simulink model "fine_delay_core"  (R2012b)
settings: Solver=ode45  StartTime=0.0  StopTime=10.0  RelTol=1e-3
libraries: xbsIndex_r4 x410, casper_library_misc x16, casper_library_multipliers x8
(part 1 of 4)
settings Model: Creator=jack  LastModifiedBy=jack

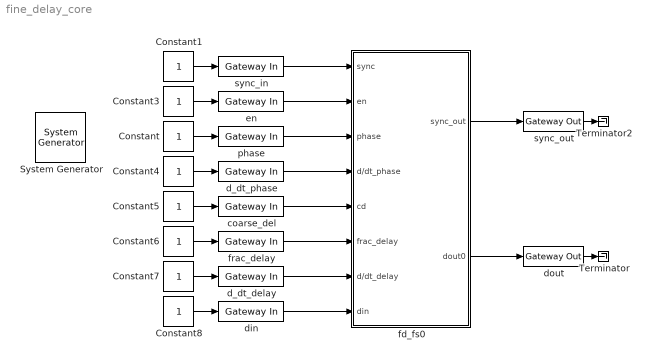
== system fine_delay_core ==
  " System Generator" : xbsIndex_r4/ System Generator  Tag=genX  xilinxfamily=virtex6  part=xc6vsx475t  speed=-1  package=ff1759  synthesis_tool=XST  clock_wrapper=Clock Enables  directory=./fine_delay_core  proj_type=Project Navigator  Synth_file=XST Defaults  Impl_file=ISE Defaults  testbench=off  simulink_period=1  sysclk_period=10  dcm_input_clock_period=10  incr_netlist=off  trim_vbits=Everywhere in SubSystem  dbl_ovrd=According to Block Masks  core_generation=According to Block Masks  run_coregen=off  deprecated_control=off  eval_field=0  block_type=sysgen
  Constant{,1,3..8} (8 alike) : Constant
  Terminator : Terminator
  Terminator2 : Terminator
  coarse_del : xbsIndex_r4/Gateway In  gui_display_data_type=Fixed-point  arith_type=Unsigned  n_bits=15  bin_pt=0  preci_type=Single  exp_width=8  frac_width=24  quantization="Round  (unbiased: +/- Inf)"  overflow=Saturate  period=1  dbl_ovrd=off  timing_constraint=None  locs_specified=off  LOCs={}  UseAsADC=off  ADCChannel='1'  inherit_from_input=off  hdl_port=on  block_type=gatewayin
  d_dt_delay : xbsIndex_r4/Gateway In  gui_display_data_type=Fixed-point  arith_type=Unsigned  n_bits=16  bin_pt=0  preci_type=Single  exp_width=8  frac_width=24  quantization="Round  (unbiased: +/- Inf)"  overflow=Saturate  period=1  dbl_ovrd=off  timing_constraint=None  locs_specified=off  LOCs={}  UseAsADC=off  ADCChannel='1'  inherit_from_input=off  hdl_port=on  block_type=gatewayin
  d_dt_phase : xbsIndex_r4/Gateway In  gui_display_data_type=Fixed-point  arith_type=Unsigned  n_bits=16  bin_pt=0  preci_type=Single  exp_width=8  frac_width=24  quantization="Round  (unbiased: +/- Inf)"  overflow=Saturate  period=1  dbl_ovrd=off  timing_constraint=None  locs_specified=off  LOCs={}  UseAsADC=off  ADCChannel='1'  inherit_from_input=off  hdl_port=on  block_type=gatewayin
  din : xbsIndex_r4/Gateway In  gui_display_data_type=Fixed-point  arith_type=Unsigned  n_bits=8*36  bin_pt=0  preci_type=Single  exp_width=8  frac_width=24  quantization="Round  (unbiased: +/- Inf)"  overflow=Saturate  period=1  dbl_ovrd=off  timing_constraint=None  locs_specified=off  LOCs={}  UseAsADC=off  ADCChannel='1'  inherit_from_input=off  hdl_port=on  block_type=gatewayin
  dout : xbsIndex_r4/Gateway Out  inherit_from_input=off  hdl_port=on  timing_constraint=None  locs_specified=off  LOCs={}  UseAsDAC=off  DACChannel='1'  block_type=gatewayout
  en : xbsIndex_r4/Gateway In  gui_display_data_type=Boolean  arith_type=Boolean  n_bits=16  bin_pt=14  preci_type=Single  exp_width=8  frac_width=24  quantization="Round  (unbiased: +/- Inf)"  overflow=Saturate  period=1  dbl_ovrd=off  timing_constraint=None  locs_specified=off  LOCs={}  UseAsADC=off  ADCChannel='1'  inherit_from_input=off  hdl_port=on  block_type=gatewayin
  fd_fs0 : Subsystem
  frac_delay : xbsIndex_r4/Gateway In  gui_display_data_type=Fixed-point  arith_type=Unsigned  n_bits=16  bin_pt=0  preci_type=Single  exp_width=8  frac_width=24  quantization="Round  (unbiased: +/- Inf)"  overflow=Saturate  period=1  dbl_ovrd=off  timing_constraint=None  locs_specified=off  LOCs={}  UseAsADC=off  ADCChannel='1'  inherit_from_input=off  hdl_port=on  block_type=gatewayin
  phase : xbsIndex_r4/Gateway In  gui_display_data_type=Fixed-point  arith_type=Unsigned  n_bits=16  bin_pt=0  preci_type=Single  exp_width=8  frac_width=24  quantization="Round  (unbiased: +/- Inf)"  overflow=Saturate  period=1  dbl_ovrd=off  timing_constraint=None  locs_specified=off  LOCs={}  UseAsADC=off  ADCChannel='1'  inherit_from_input=off  hdl_port=on  block_type=gatewayin
  sync_in : xbsIndex_r4/Gateway In  gui_display_data_type=Boolean  arith_type=Boolean  n_bits=16  bin_pt=14  preci_type=Single  exp_width=8  frac_width=24  quantization="Round  (unbiased: +/- Inf)"  overflow=Saturate  period=1  dbl_ovrd=off  timing_constraint=None  locs_specified=off  LOCs={}  UseAsADC=off  ADCChannel='1'  inherit_from_input=off  hdl_port=on  block_type=gatewayin
  sync_out : xbsIndex_r4/Gateway Out  inherit_from_input=off  hdl_port=on  timing_constraint=None  locs_specified=off  LOCs={}  UseAsDAC=off  DACChannel='1'  block_type=gatewayout
  wires:
  fd_fs0/1(sync_out) -> sync_out/1
  fd_fs0/2(dout0) -> dout/1
  sync_in/1 -> fd_fs0/1(sync)
  Constant/1 -> phase/1
  Constant1/1 -> sync_in/1
  dout/1 -> Terminator/1
  sync_out/1 -> Terminator2/1
  Constant3/1 -> en/1
  en/1 -> fd_fs0/2(en)
  phase/1 -> fd_fs0/3(phase)
  Constant4/1 -> d_dt_phase/1
  d_dt_phase/1 -> fd_fs0/4(d/dt_phase)
  Constant6/1 -> frac_delay/1
  Constant8/1 -> din/1
  Constant7/1 -> d_dt_delay/1
  Constant5/1 -> coarse_del/1
  din/1 -> fd_fs0/8(din)
  d_dt_delay/1 -> fd_fs0/7(d/dt_delay)
  coarse_del/1 -> fd_fs0/5(cd)
  frac_delay/1 -> fd_fs0/6(frac_delay)

== system fine_delay_core/fd_fs0 ==
  sync : Inport
  en : Inport  Port=2
  phase : Inport  Port=3
  d/dt_phase : Inport  Port=4
  cd : Inport  Port=5
  frac_delay : Inport  Port=6
  d/dt_delay : Inport  Port=7
  din : Inport  Port=8
  Concat : xbsIndex_r4/Concat  num_inputs=2  dbl_ovrd=off  block_type=concat
  Constant53 : xbsIndex_r4/Constant  const=0  gui_display_data_type=Fixed-point  arith_type=Boolean  n_bits=1  bin_pt=0  preci_type=Single  exp_width=8  frac_width=24  explicit_period=off  period=1  equ=P=C  opselect=C  inp2=PCIN>>17  opr=+  inp1=P  carry=CIN  dbl_ovrd=off  block_type=constant
      settings: block_version=11.4
  Terminator59 : Terminator
  Terminator60 : Terminator
  delay_gen0 : Subsystem  mask{fft_len=12, phase_bits=16, max_fringe_rate=23, min_fringe_rate=38, delay_bits=16+15, delay_bin_pt=16, max_delay_rate=23, min_delay_rate=38, add_latency=1, lookup_bits=11, cd_bits=15}
      mask prompts: fft_len "FFT size (2^?)"; phase_bits "Input phase resolution (2*pi/2^? radians)"; max_fringe_rate "Max fringe update rate (1/2^? radians/sample)"; min_fringe_rate "Min (non-zero) fringe rate (1/2^? radians/sample)"; delay_bits "Input delay resolution (bits)"; delay_bin_pt "Input delay binary point"; max_delay_rate "Max delay update rate (1/2^? samples/sample)"; min_delay_rate "Min (non-zero) delay update rate (1/2^? samples/sample)"; add_latency "Add latency"; lookup_bits "DDS lookup table resolution (2*pi/2^?)"; cd_bits "Coarse delay range (2^? bits)"
  fd_fs0 : Subsystem  mask{lookup_bit_width=11, data_bit_width=18, fft_len=10, mix_bits=18, bram_latency=3, mult_latency=2, add_latency=1, conv_latency=3}
      mask prompts: lookup_bit_width "Phase resolution (2pi/2^?)"; data_bit_width "Data bit width"; fft_len "FFT length 2^?"; mix_bits "Mixing product bit width"; bram_latency "BRAM latency"; mult_latency "Mult latency"; add_latency "Adder latency"; conv_latency "Convert latency"
      mask init:
      | for i=[0:7]
      |     set_param([gcb,'/rotate',num2str(i),'/sincos0'], ...
      |         'bit_width', 'mix_bits', ...
      |         'bram_latency', 'bram_latency', ...
      |         'depth_bits', 'lookup_bit_width');
      | end
  sync_out : Outport
  dout0 : Outport  Port=2
  wires:
  fd_fs0/1(sync_out) -> sync_out/1
  delay_gen0/3(cd_o) -> Terminator60/1
  delay_gen0/2(en_out) -> Terminator59/1
  delay_gen0/5(slope_out) -> fd_fs0/3(a1)
  delay_gen0/4(phase_out) -> fd_fs0/2(a0)
  delay_gen0/1(sync_out) -> fd_fs0/1(sync_in)
  sync/1 -> delay_gen0/1(sync_in)
  en/1 -> delay_gen0/2(en)
  phase/1 -> delay_gen0/3(phase)
  d/dt_phase/1 -> delay_gen0/4(d/dt_phase)
  din/1 -> delay_gen0/7(din)
  d/dt_delay/1 -> delay_gen0/6(d/dt_delay)
  cd/1 -> Concat/1
  frac_delay/1 -> Concat/2
  Concat/1 -> delay_gen0/5(delay)
  Constant53/1 -> delay_gen0/8(invert_slope)
  delay_gen0/6(dout) -> fd_fs0/4(din)
  delay_gen0/7(idx_d0) -> fd_fs0/5(idx_din0)
  delay_gen0/8(idx_d1) -> fd_fs0/6(idx_din1)
  delay_gen0/9(idx_d2) -> fd_fs0/7(idx_din2)
  delay_gen0/10(idx_d3) -> fd_fs0/8(idx_din3)
  delay_gen0/11(idx_d4) -> fd_fs0/9(idx_din4)
  delay_gen0/12(idx_d5) -> fd_fs0/10(idx_din5)
  delay_gen0/13(idx_d6) -> fd_fs0/11(idx_din6)
  delay_gen0/14(idx_d7) -> fd_fs0/12(idx_din7)
  fd_fs0/2(dout) -> dout0/1

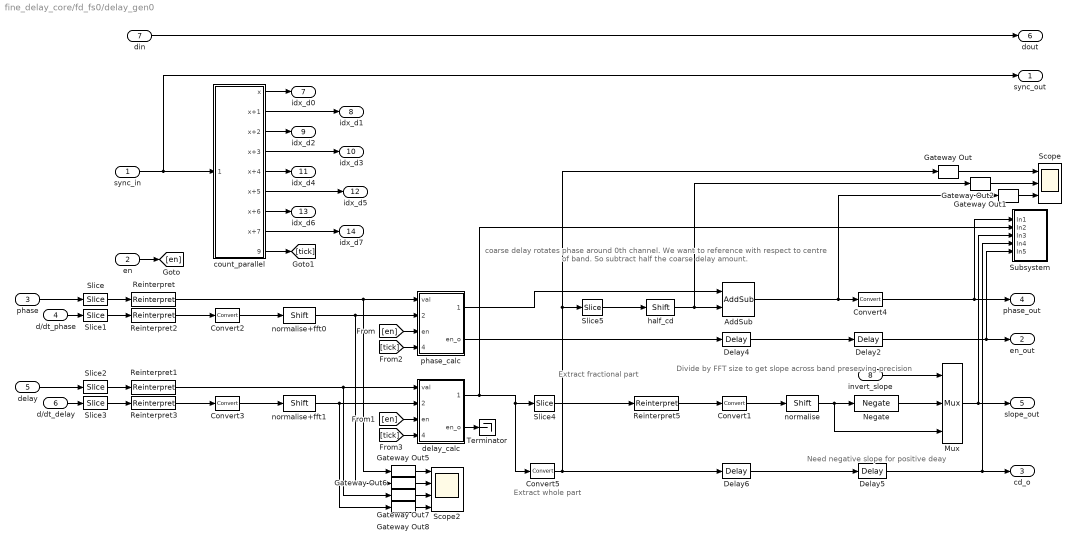
== system fine_delay_core/fd_fs0/delay_gen0 ==
  note: Need negative slope
      | for positive deay
  note: Divide by FFT size
      | to get slope
      | across band
      | preserving precision
  note: Extract whole part
  note: Extract fractional part
  note: coarse delay rotates phase around 0th
      | channel. We want to reference with respect to
      | centre of band. So subtract half the coarse
      | delay amount.
  sync_in : Inport
  en : Inport  Port=2
  phase : Inport  Port=3
  d/dt_phase : Inport  Port=4
  delay : Inport  Port=5
  d/dt_delay : Inport  Port=6
  din : Inport  Port=7
  invert_slope : Inport  Port=8
  AddSub : xbsIndex_r4/AddSub  mode=Addition  use_carryin=off  use_carryout=off  en=off  latency=0  precision=Full  arith_type=Unsigned  n_bits=16  bin_pt=14  quantization=Truncate  overflow=Wrap  dbl_ovrd=off  use_behavioral_HDL=off  hw_selection=Fabric  pipelined=off  block_type=addsub
  Convert1 : xbsIndex_r4/Convert  gui_display_data_type=Fixed-point  arith_type="Signed  (2's comp)"  n_bits=lookup_bits + fft_len  bin_pt=lookup_bits + fft_len -1  float_type=Single  exp_bits=8  fraction_bits=24  quantization="Round  (unbiased: +/- Inf)"  overflow=Wrap  en=off  latency=1  dbl_ovrd=off  pipeline=on  block_type=convert
      settings: block_version=10.1.3
  Convert2 : xbsIndex_r4/Convert  gui_display_data_type=Fixed-point  arith_type="Signed  (2's comp)"  n_bits=min_fringe_rate-fft_len+1  bin_pt=min_fringe_rate-fft_len  float_type=Single  exp_bits=8  fraction_bits=24  quantization=Truncate  overflow=Wrap  en=off  latency=0  dbl_ovrd=off  pipeline=on  block_type=convert
      settings: block_version=10.1.3
  Convert3 : xbsIndex_r4/Convert  gui_display_data_type=Fixed-point  arith_type="Signed  (2's comp)"  n_bits=min_delay_rate-fft_len+1  bin_pt=min_delay_rate-fft_len  float_type=Single  exp_bits=8  fraction_bits=24  quantization=Truncate  overflow=Wrap  en=off  latency=0  dbl_ovrd=off  pipeline=on  block_type=convert
      settings: block_version=10.1.3
  Convert4 : xbsIndex_r4/Convert  gui_display_data_type=Fixed-point  arith_type="Signed  (2's comp)"  n_bits=max(phase_bits, min_fringe_rate-fft_len+1)  bin_pt=max(phase_bits-1, min_fringe_rate-fft_len)  float_type=Single  exp_bits=8  fraction_bits=24  quantization=Truncate  overflow=Wrap  en=off  latency=0  dbl_ovrd=off  pipeline=on  block_type=convert
      settings: block_version=10.1.3
  Convert5 : xbsIndex_r4/Convert  gui_display_data_type=Fixed-point  arith_type=Unsigned  n_bits=cd_bits  bin_pt=0  float_type=Single  exp_bits=8  fraction_bits=24  quantization=Truncate  overflow=Wrap  en=off  latency=0  dbl_ovrd=off  pipeline=on  block_type=convert
      settings: block_version=10.1.3
  Delay{2,4..6} (4 alike) : xbsIndex_r4/Delay  rst=off  infoeditControl=Selection of Reset will increase slice count due to use of real FFs and instead of SRLs  en=off  latency=1  dbl_ovrd=off  reg_retiming=on  block_type=delay
      settings: block_version=11.4
  Gateway Out{,1..2,5..8} (7 alike) : xbsIndex_r4/Gateway Out  inherit_from_input=off  hdl_port=off  timing_constraint=None  locs_specified=off  LOCs={}  UseAsDAC=off  DACChannel='1'  block_type=gatewayout
      settings: infoedit="Gateway out block.  Converts Xilinx fixed point inputs into ouputs of type Simulink integer, double, or fixed point.<br><br>Hardware notes:  In hardware these blocks become top level output ports or are discarded, depending on how they are configured."  block_version=11.4
  Mux : xbsIndex_r4/Mux  inputs=2  en=off  latency=0  precision=Full  arith_type=Unsigned  n_bits=16  bin_pt=14  quantization=Truncate  overflow=Wrap  dbl_ovrd=off  block_type=mux
      settings: block_version=11.4
  Negate : xbsIndex_r4/Negate  precision=User Defined  arith_type="Signed  (2's comp)"  n_bits=lookup_bits + fft_len  bin_pt=lookup_bits + fft_len - 1  quantization=Truncate  overflow=Wrap  en=off  latency=1  dbl_ovrd=off  block_type=negate
      settings: block_version=11.4
  Reinterpret : xbsIndex_r4/Reinterpret  force_arith_type=on  arith_type="Signed  (2's comp)"  force_bin_pt=on  bin_pt=phase_bits-1  block_type=reinterpret
      settings: infoedit="Changes signal type without altering the binary representation.   You can changed the signal between signed and unsigned, and relocate the binary point.<br><br>Hardware notes: In hardware this block costs nothing.<br><br>Example:  Suppose the input is 6 bits wide, signed, with 2 fractional bits, and the output is forced to unsigned with 0 fractional bits.  Then an input of -2.0 (1110.00 in binary 2's complement) becomes an output of 56 (111000 in binary)."
  Reinterpret1 : xbsIndex_r4/Reinterpret  force_arith_type=on  arith_type=Unsigned  force_bin_pt=on  bin_pt=delay_bin_pt  block_type=reinterpret
      settings: infoedit="Changes signal type without altering the binary representation.   You can changed the signal between signed and unsigned, and relocate the binary point.<br><br>Hardware notes: In hardware this block costs nothing.<br><br>Example:  Suppose the input is 6 bits wide, signed, with 2 fractional bits, and the output is forced to unsigned with 0 fractional bits.  Then an input of -2.0 (1110.00 in binary 2's complement) becomes an output of 56 (111000 in binary)."
  Reinterpret2 : xbsIndex_r4/Reinterpret  force_arith_type=on  arith_type="Signed  (2's comp)"  force_bin_pt=on  bin_pt=min_fringe_rate-max_fringe_rate  block_type=reinterpret
      settings: infoedit="Changes signal type without altering the binary representation.   You can changed the signal between signed and unsigned, and relocate the binary point.<br><br>Hardware notes: In hardware this block costs nothing.<br><br>Example:  Suppose the input is 6 bits wide, signed, with 2 fractional bits, and the output is forced to unsigned with 0 fractional bits.  Then an input of -2.0 (1110.00 in binary 2's complement) becomes an output of 56 (111000 in binary)."
  Reinterpret3 : xbsIndex_r4/Reinterpret  force_arith_type=on  arith_type="Signed  (2's comp)"  force_bin_pt=on  bin_pt=min_delay_rate-max_delay_rate  block_type=reinterpret
      settings: infoedit="Changes signal type without altering the binary representation.   You can changed the signal between signed and unsigned, and relocate the binary point.<br><br>Hardware notes: In hardware this block costs nothing.<br><br>Example:  Suppose the input is 6 bits wide, signed, with 2 fractional bits, and the output is forced to unsigned with 0 fractional bits.  Then an input of -2.0 (1110.00 in binary 2's complement) becomes an output of 56 (111000 in binary)."
  Reinterpret5 : xbsIndex_r4/Reinterpret  force_arith_type=on  arith_type=Unsigned  force_bin_pt=on  bin_pt=max(delay_bin_pt-1, min_delay_rate-fft_len)  block_type=reinterpret
      settings: infoedit="Changes signal type without altering the binary representation.   You can changed the signal between signed and unsigned, and relocate the binary point.<br><br>Hardware notes: In hardware this block costs nothing.<br><br>Example:  Suppose the input is 6 bits wide, signed, with 2 fractional bits, and the output is forced to unsigned with 0 fractional bits.  Then an input of -2.0 (1110.00 in binary 2's complement) becomes an output of 56 (111000 in binary)."
  Scope : Scope  NumInputPorts=3
      settings: YMin=2~1~1  YMax=2~1~1
  Scope2 : Scope  NumInputPorts=4
      settings: YMin=-5~-5~-5~-5  YMax=5~5~5~5  SaveName=ScopeData6
  Slice : xbsIndex_r4/Slice  nbits=phase_bits  boolean_output=off  mode=Lower Bit Location + Width  bit1=0  base1=MSB of Input  bit0=0  base0=LSB of Input  dbl_ovrd=off  block_type=slice
  Slice1 : xbsIndex_r4/Slice  nbits=min_fringe_rate-max_fringe_rate+1  boolean_output=off  mode=Lower Bit Location + Width  bit1=0  base1=MSB of Input  bit0=0  base0=LSB of Input  dbl_ovrd=off  block_type=slice
  Slice2 : xbsIndex_r4/Slice  nbits=delay_bits  boolean_output=off  mode=Lower Bit Location + Width  bit1=0  base1=MSB of Input  bit0=0  base0=LSB of Input  dbl_ovrd=off  block_type=slice
  Slice3 : xbsIndex_r4/Slice  nbits=min_delay_rate-max_delay_rate+1  boolean_output=off  mode=Lower Bit Location + Width  bit1=0  base1=MSB of Input  bit0=0  base0=LSB of Input  dbl_ovrd=off  block_type=slice
  Slice4 : xbsIndex_r4/Slice  nbits=max(delay_bin_pt-1, min_delay_rate-fft_len)  boolean_output=off  mode=Lower Bit Location + Width  bit1=0  base1=MSB of Input  bit0=0  base0=LSB of Input  dbl_ovrd=off  block_type=slice
  Slice5 : xbsIndex_r4/Slice  nbits=2  boolean_output=off  mode=Lower Bit Location + Width  bit1=0  base1=MSB of Input  bit0=0  base0=LSB of Input  dbl_ovrd=off  block_type=slice
  Subsystem : Subsystem
  Terminator : Terminator
  count_parallel : Subsystem  mask{outputs=3, period=fft_len, delay=2+2+1}
      mask prompts: outputs "Number of parallel outputs (2^?)"; period "Period of counter (2^?)"; delay "Delay to compensate for"
  delay_calc : Subsystem  mask{bit_width=max(delay_bits, min_delay_rate-fft_len+cd_bits), bin_pt=max(delay_bin_pt-1, min_delay_rate-fft_len)}
      mask prompts: bit_width "Coefficient bit width"; bin_pt "Coefficient binary point"
  half_cd : xbsIndex_r4/Shift  shift_dir=Right  shift_bits=1  en=off  latency=0  precision=User Defined  arith_type=Unsigned  n_bits=2  bin_pt=1  quantization=Truncate  overflow=Saturate  dbl_ovrd=off  block_type=shift
  normalise : xbsIndex_r4/Shift  shift_dir=Right  shift_bits=fft_len  en=off  latency=0  precision=Full  arith_type="Signed  (2's comp)"  n_bits=max(delay_bits-1, min_delay_rate-fft_len) + fft_len  bin_pt=max(delay_bits-1, min_delay_rate-fft_len) + fft_len -1  quantization=Truncate  overflow=Wrap  dbl_ovrd=off  block_type=shift
  normalise+fft0 : xbsIndex_r4/Shift  shift_dir=Right  shift_bits=max_fringe_rate-fft_len  en=off  latency=0  precision=Full  arith_type="Signed  (2's comp)"  n_bits=16  bin_pt=14  quantization=Truncate  overflow=Wrap  dbl_ovrd=off  block_type=shift
  normalise+fft1 : xbsIndex_r4/Shift  shift_dir=Right  shift_bits=max_delay_rate-fft_len  en=off  latency=0  precision=Full  arith_type="Signed  (2's comp)"  n_bits=16  bin_pt=14  quantization=Truncate  overflow=Wrap  dbl_ovrd=off  block_type=shift
  phase_calc : Subsystem  mask{bit_width=max(phase_bits, min_fringe_rate-fft_len+1), bin_pt=max(phase_bits-1, min_fringe_rate-fft_len)}
      mask prompts: bit_width "Coefficient bit width"; bin_pt "Coefficient binary point"
  sync_out : Outport
  en_out : Outport  Port=2
  cd_o : Outport  Port=3
  phase_out : Outport  Port=4
  slope_out : Outport  Port=5
  dout : Outport  Port=6
  idx_d0 : Outport  Port=7
  idx_d1 : Outport  Port=8
  idx_d2 : Outport  Port=9
  idx_d3 : Outport  Port=10
  idx_d4 : Outport  Port=11
  idx_d5 : Outport  Port=12
  idx_d6 : Outport  Port=13
  idx_d7 : Outport  Port=14
  wires:
  Delay5/1 -> cd_o/1, Subsystem/4(In4)
  Delay2/1 -> en_out/1, Subsystem/5(In5)
  Convert4/1 -> phase_out/1, Subsystem/1(In1)
  Mux/1 -> slope_out/1, Subsystem/3(In3)
  normalise/1 -> Mux/3, Negate/1
  delay_calc/2(en_o) -> Terminator/1
  Convert1/1 -> normalise/1
  phase_calc/2(en_o) -> Delay4/1
  delay_calc/1(coeff) -> Subsystem/2(In2), Slice4/1, Convert5/1
  [tick] -> delay_calc/4(update)
  [tick] -> phase_calc/4(update)
  [en] -> delay_calc/3(en)
  [en] -> phase_calc/3(en)
  Reinterpret3/1 -> Convert3/1
  Reinterpret2/1 -> Convert2/1
  Reinterpret1/1 -> delay_calc/1(val), Gateway Out7/1
  Reinterpret/1 -> phase_calc/1(val), Gateway Out5/1
  Slice3/1 -> Reinterpret3/1
  Slice2/1 -> Reinterpret1/1
  Slice1/1 -> Reinterpret2/1
  Slice/1 -> Reinterpret/1
  din/1 -> dout/1
  normalise+fft0/1 -> phase_calc/2(val_inc), Gateway Out6/1
  Convert2/1 -> normalise+fft0/1
  normalise+fft1/1 -> delay_calc/2(val_inc), Gateway Out8/1
  Convert3/1 -> normalise+fft1/1
  d/dt_delay/1 -> Slice3/1
  delay/1 -> Slice2/1
  d/dt_phase/1 -> Slice1/1
  phase/1 -> Slice/1
  Gateway Out8/1 -> Scope2/4
  Gateway Out7/1 -> Scope2/3
  Gateway Out6/1 -> Scope2/2
  Gateway Out5/1 -> Scope2/1
  count_parallel/2(x+1) -> idx_d1/1
  count_parallel/1(x) -> idx_d0/1
  en/1 -> [en]
  sync_in/1 -> count_parallel/1(sync_in), sync_out/1
  AddSub/1 -> Convert4/1, Gateway Out2/1
  Delay4/1 -> Delay2/1
  Slice4/1 -> Reinterpret5/1
  invert_slope/1 -> Mux/1
  Negate/1 -> Mux/2
  Reinterpret5/1 -> Convert1/1
  Convert5/1 -> Delay6/1, Slice5/1, Gateway Out/1
  Delay6/1 -> Delay5/1
  Slice5/1 -> half_cd/1
  phase_calc/1(coeff) -> AddSub/1
  half_cd/1 -> AddSub/2, Gateway Out1/1
  Gateway Out/1 -> Scope/1
  Gateway Out1/1 -> Scope/2
  Gateway Out2/1 -> Scope/3
  count_parallel/3(x+2) -> idx_d2/1
  count_parallel/4(x+3) -> idx_d3/1
  count_parallel/5(x+4) -> idx_d4/1
  count_parallel/6(x+5) -> idx_d5/1
  count_parallel/7(x+6) -> idx_d6/1
  count_parallel/8(x+7) -> idx_d7/1
  count_parallel/9(update) -> [tick]

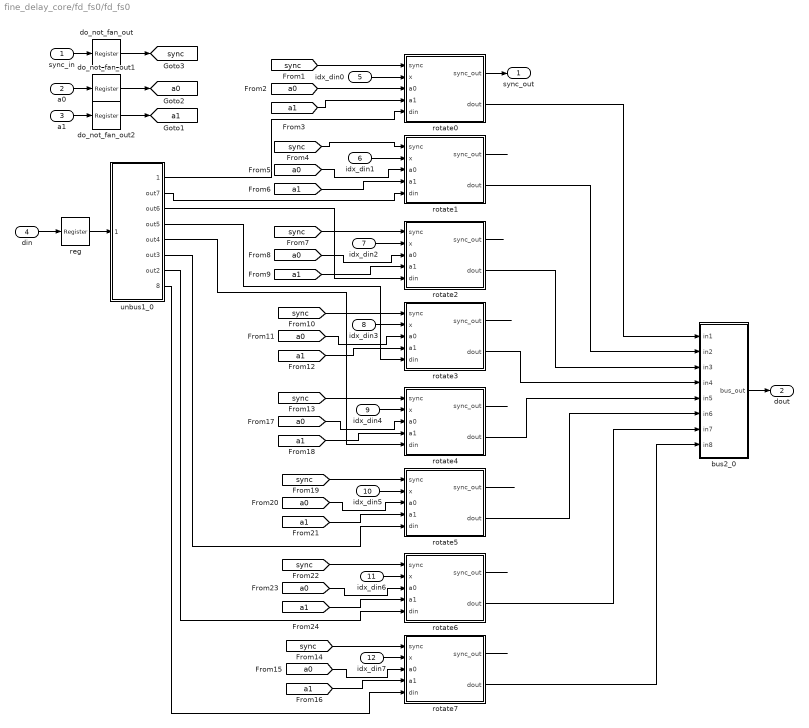
== system fine_delay_core/fd_fs0/fd_fs0 ==
  sync_in : Inport
  a0 : Inport  Port=2
  a1 : Inport  Port=3
  din : Inport  Port=4
  idx_din0 : Inport  Port=5
  idx_din1 : Inport  Port=6
  idx_din2 : Inport  Port=7
  idx_din3 : Inport  Port=8
  idx_din4 : Inport  Port=9
  idx_din5 : Inport  Port=10
  idx_din6 : Inport  Port=11
  idx_din7 : Inport  Port=12
  bus2_0 : Subsystem  AncestorBlock=casper_library_flow_control/bus_create  mask(bus_create){inputNum=8}
      mask prompts: inputNum "Number of inputs:"
      mask init:
      | bus_create_init(gcb,...
      |     'inputNum', inputNum);
  do_not_fan_out : xbsIndex_r4/Register  init=0  rst=off  en=off  dbl_ovrd=off  block_type=register
  do_not_fan_out1 : xbsIndex_r4/Register  init=0  rst=off  en=off  dbl_ovrd=off  block_type=register
  do_not_fan_out2 : xbsIndex_r4/Register  init=0  rst=off  en=off  dbl_ovrd=off  block_type=register
  reg : xbsIndex_r4/Register  init=0  rst=off  en=off  dbl_ovrd=off  block_type=register
  rotate0 : Subsystem  mask{lookup_bit_width=lookup_bit_width, data_bit_width=data_bit_width, fft_len=fft_len, mix_bits=mix_bits, bram_latency=bram_latency, mult_latency=mult_latency, add_latency=add_latency, conv_latency=conv_latency}
      mask prompts: lookup_bit_width "Phase resolution"; data_bit_width "Data bit width"; fft_len "FFT length (2^?)"; mix_bits "Mixing product bit width"; bram_latency "BRAM latency"; mult_latency "Multiplier latency"; add_latency "Adder latency"; conv_latency "Convert latency"
  rotate1 : Subsystem  mask{lookup_bit_width=lookup_bit_width, data_bit_width=data_bit_width, fft_len=fft_len, mix_bits=mix_bits, bram_latency=bram_latency, mult_latency=mult_latency, add_latency=add_latency, conv_latency=conv_latency}
      mask prompts: lookup_bit_width "Phase resolution"; data_bit_width "Data bit width"; fft_len "FFT length (2^?)"; mix_bits "Mixing product bit width"; bram_latency "BRAM latency"; mult_latency "Multiplier latency"; add_latency "Adder latency"; conv_latency "Convert latency"
  rotate2 : Subsystem  mask{lookup_bit_width=lookup_bit_width, data_bit_width=data_bit_width, fft_len=fft_len, mix_bits=mix_bits, bram_latency=bram_latency, mult_latency=mult_latency, add_latency=add_latency, conv_latency=conv_latency}
      mask prompts: lookup_bit_width "Phase resolution"; data_bit_width "Data bit width"; fft_len "FFT length (2^?)"; mix_bits "Mixing product bit width"; bram_latency "BRAM latency"; mult_latency "Multiplier latency"; add_latency "Adder latency"; conv_latency "Convert latency"
  rotate3 : Subsystem  mask{lookup_bit_width=lookup_bit_width, data_bit_width=data_bit_width, fft_len=fft_len, mix_bits=mix_bits, bram_latency=bram_latency, mult_latency=mult_latency, add_latency=add_latency, conv_latency=conv_latency}
      mask prompts: lookup_bit_width "Phase resolution"; data_bit_width "Data bit width"; fft_len "FFT length (2^?)"; mix_bits "Mixing product bit width"; bram_latency "BRAM latency"; mult_latency "Multiplier latency"; add_latency "Adder latency"; conv_latency "Convert latency"
  rotate4 : Subsystem  mask{lookup_bit_width=lookup_bit_width, data_bit_width=data_bit_width, fft_len=fft_len, mix_bits=mix_bits, bram_latency=bram_latency, mult_latency=mult_latency, add_latency=add_latency, conv_latency=conv_latency}
      mask prompts: lookup_bit_width "Phase resolution"; data_bit_width "Data bit width"; fft_len "FFT length (2^?)"; mix_bits "Mixing product bit width"; bram_latency "BRAM latency"; mult_latency "Multiplier latency"; add_latency "Adder latency"; conv_latency "Convert latency"
  rotate5 : Subsystem  mask{lookup_bit_width=lookup_bit_width, data_bit_width=data_bit_width, fft_len=fft_len, mix_bits=mix_bits, bram_latency=bram_latency, mult_latency=mult_latency, add_latency=add_latency, conv_latency=conv_latency}
      mask prompts: lookup_bit_width "Phase resolution"; data_bit_width "Data bit width"; fft_len "FFT length (2^?)"; mix_bits "Mixing product bit width"; bram_latency "BRAM latency"; mult_latency "Multiplier latency"; add_latency "Adder latency"; conv_latency "Convert latency"
  rotate6 : Subsystem  mask{lookup_bit_width=lookup_bit_width, data_bit_width=data_bit_width, fft_len=fft_len, mix_bits=mix_bits, bram_latency=bram_latency, mult_latency=mult_latency, add_latency=add_latency, conv_latency=conv_latency}
      mask prompts: lookup_bit_width "Phase resolution"; data_bit_width "Data bit width"; fft_len "FFT length (2^?)"; mix_bits "Mixing product bit width"; bram_latency "BRAM latency"; mult_latency "Multiplier latency"; add_latency "Adder latency"; conv_latency "Convert latency"
  rotate7 : Subsystem  mask{lookup_bit_width=lookup_bit_width, data_bit_width=data_bit_width, fft_len=fft_len, mix_bits=mix_bits, bram_latency=bram_latency, mult_latency=mult_latency, add_latency=add_latency, conv_latency=conv_latency}
      mask prompts: lookup_bit_width "Phase resolution"; data_bit_width "Data bit width"; fft_len "FFT length (2^?)"; mix_bits "Mixing product bit width"; bram_latency "BRAM latency"; mult_latency "Multiplier latency"; add_latency "Adder latency"; conv_latency "Convert latency"
  unbus1_0 : Subsystem  AncestorBlock=casper_library_flow_control/bus_expand  mask(bus_expand){mode=divisions of equal size, outputNum=8, outputWidth=36, outputBinaryPt=0, outputArithmeticType=0, show_format=off, outputToWorkspace=off, variablePrefix=out, outputToModelAsWell=on}
      mask prompts: outputNum "Number of outputs:"; outputWidth "Output width:"; outputBinaryPt "Output binary point position:"; outputArithmeticType "Output arithmetic type (ufix=0, fix=1, bool=2):"; show_format "Print format string?"; outputToWorkspace "Output to workspace?"; variablePrefix "Variable name prefix:"; outputToModelAsWell "Output to model as well?"
      mask help:
      | Expands a 'bus' made using a bus_create or Xilinx
      | concat block.
      | The input will be divided into the specified number
      | of outputs with the specified arithmetic types.
      | Divisions are made from most significant bit.
      mask init:
      | bus_expand_init(gcb,...
      |     'mode', mode, ...
      |     'outputNum', outputNum, ...
      |     'outputWidth', outputWidth, ...
      |     'outputBinaryPt', outputBinaryPt, ...
      |     'outputArithmeticType', outputArithmeticType, ...
      |     'show_format', show_format, ...
      |     'outputToWorkspace', outputToWorkspace, ...
      |     'variablePrefix', variablePrefix, ...
      |     'outputToModelAsWell', outputToModelAsWell);
      settings: AttributesFormatString=8 outputs
      mask TypeOptions mode: divisions of equal size | divisions of arbitrary size
      mask Callback mode: bus_expand_callback();
      mask Callback outputWidth: bus_expand_callback();
      mask Callback outputToWorkspace: bus_expand_callback();
  sync_out : Outport
  dout : Outport  Port=2
  tag scope: a0=global, a1=global, sync=global
  wires:
  rotate0/1(sync_out) -> sync_out/1
  idx_din0/1 -> rotate0/2(x)
  sync_in/1 -> do_not_fan_out/1
  a0/1 -> do_not_fan_out1/1
  a1/1 -> do_not_fan_out2/1
  [sync] -> rotate0/1(sync)
  [a0] -> rotate0/3(a0)
  [a1] -> rotate0/4(a1)
  rotate1/1(sync_out) -> ?
  idx_din1/1 -> rotate1/2(x)
  [sync] -> rotate1/1(sync)
  [a0] -> rotate1/3(a0)
  [a1] -> rotate1/4(a1)
  idx_din2/1 -> rotate2/2(x)
  [sync] -> rotate2/1(sync)
  [a0] -> rotate2/3(a0)
  [a1] -> rotate2/4(a1)
  rotate3/1(sync_out) -> ?
  idx_din3/1 -> rotate3/2(x)
  [sync] -> rotate3/1(sync)
  [a0] -> rotate3/3(a0)
  [a1] -> rotate3/4(a1)
  rotate4/1(sync_out) -> ?
  idx_din4/1 -> rotate4/2(x)
  [sync] -> rotate4/1(sync)
  [a0] -> rotate4/3(a0)
  [a1] -> rotate4/4(a1)
  rotate5/1(sync_out) -> ?
  idx_din5/1 -> rotate5/2(x)
  [sync] -> rotate5/1(sync)
  [a0] -> rotate5/3(a0)
  [a1] -> rotate5/4(a1)
  idx_din6/1 -> rotate6/2(x)
  [sync] -> rotate6/1(sync)
  [a0] -> rotate6/3(a0)
  [a1] -> rotate6/4(a1)
  rotate7/1(sync_out) -> ?
  idx_din7/1 -> rotate7/2(x)
  [sync] -> rotate7/1(sync)
  [a0] -> rotate7/3(a0)
  [a1] -> rotate7/4(a1)
  din/1 -> reg/1
  unbus1_0/1(msb_out8) -> rotate0/5(din)
  unbus1_0/2(out7) -> rotate1/5(din)
  unbus1_0/3(out6) -> rotate2/5(din)
  unbus1_0/4(out5) -> rotate3/5(din)
  unbus1_0/5(out4) -> rotate4/5(din)
  unbus1_0/6(out3) -> rotate5/5(din)
  unbus1_0/7(out2) -> rotate6/5(din)
  unbus1_0/8(lsb_out1) -> rotate7/5(din)
  bus2_0/1(bus_out) -> dout/1
  rotate0/2(dout) -> bus2_0/1(in1)
  rotate1/2(dout) -> bus2_0/2(in2)
  rotate2/2(dout) -> bus2_0/3(in3)
  rotate3/2(dout) -> bus2_0/4(in4)
  rotate4/2(dout) -> bus2_0/5(in5)
  rotate5/2(dout) -> bus2_0/6(in6)
  rotate6/2(dout) -> bus2_0/7(in7)
  rotate7/2(dout) -> bus2_0/8(in8)
  rotate2/1(sync_out) -> ?
  rotate6/1(sync_out) -> ?
  do_not_fan_out/1 -> [sync]
  do_not_fan_out1/1 -> [a0]
  do_not_fan_out2/1 -> [a1]
  reg/1 -> unbus1_0/1(bus_in)

== system fine_delay_core/fd_fs0/delay_gen0/Subsystem ==
  In1 : Inport
  In2 : Inport  Port=2
  In3 : Inport  Port=3
  In4 : Inport  Port=4
  In5 : Inport  Port=5
  Delay4 : xbsIndex_r4/Delay  rst=off  infoeditControl=Selection of Reset will increase slice count due to use of real FFs and instead of SRLs  en=off  latency=1  dbl_ovrd=off  reg_retiming=on  block_type=delay
      settings: block_version=11.4
  Disregard Subsystem : xbsIndex_r4/Disregard Subsystem  Tag=discardX  block_type=disregard
      settings: block_version=11.4
  Gateway Out{,1..4} (5 alike) : xbsIndex_r4/Gateway Out  inherit_from_input=off  hdl_port=off  timing_constraint=None  locs_specified=off  LOCs={}  UseAsDAC=off  DACChannel='1'  block_type=gatewayout
      settings: infoedit="Gateway out block.  Converts Xilinx fixed point inputs into ouputs of type Simulink integer, double, or fixed point.<br><br>Hardware notes:  In hardware these blocks become top level output ports or are discarded, depending on how they are configured."  block_version=11.4
  Scope : Scope  NumInputPorts=5
      settings: TimeRange=50000  YMin=-0.5~1~-1~1~0  YMax=-0.5~1~1~1~1  SaveName=ScopeData3
  wires:
  Delay4/1 -> Gateway Out1/1
  Gateway Out4/1 -> Scope/5
  Gateway Out3/1 -> Scope/4
  Gateway Out2/1 -> Scope/3
  Gateway Out1/1 -> Scope/2
  Gateway Out/1 -> Scope/1
  In1/1 -> Gateway Out/1
  In2/1 -> Delay4/1
  In3/1 -> Gateway Out2/1
  In4/1 -> Gateway Out3/1
  In5/1 -> Gateway Out4/1

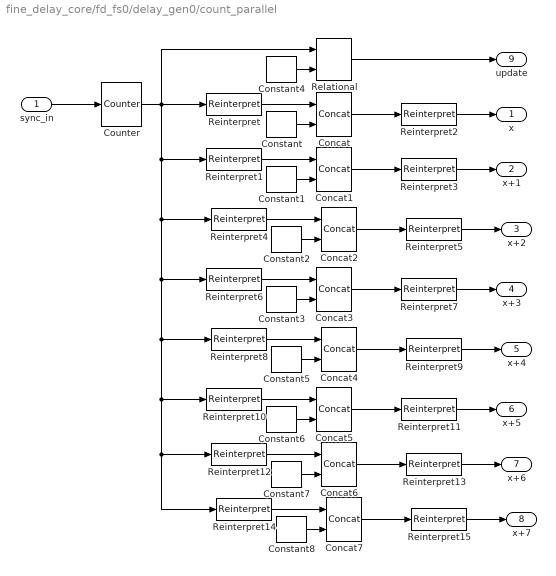
== system fine_delay_core/fd_fs0/delay_gen0/count_parallel ==
  sync_in : Inport
  Concat{,1..7} (8 alike) : xbsIndex_r4/Concat  num_inputs=2  dbl_ovrd=off  block_type=concat
      settings: block_version=10.1.3
  Constant : xbsIndex_r4/Constant  const=0  gui_display_data_type=Fixed-point  arith_type=Unsigned  n_bits=outputs  bin_pt=0  preci_type=Single  exp_width=8  frac_width=24  explicit_period=off  period=1  equ=P=C  opselect=C  inp2=PCIN>>17  opr=+  inp1=P  carry=CIN  dbl_ovrd=off  block_type=constant
  Constant1 : xbsIndex_r4/Constant  const=1  gui_display_data_type=Fixed-point  arith_type=Unsigned  n_bits=outputs  bin_pt=0  preci_type=Single  exp_width=8  frac_width=24  explicit_period=off  period=1  equ=P=C  opselect=C  inp2=PCIN>>17  opr=+  inp1=P  carry=CIN  dbl_ovrd=off  block_type=constant
  Constant2 : xbsIndex_r4/Constant  const=2  gui_display_data_type=Fixed-point  arith_type=Unsigned  n_bits=outputs  bin_pt=0  preci_type=Single  exp_width=8  frac_width=24  explicit_period=off  period=1  equ=P=C  opselect=C  inp2=PCIN>>17  opr=+  inp1=P  carry=CIN  dbl_ovrd=off  block_type=constant
  Constant3 : xbsIndex_r4/Constant  const=3  gui_display_data_type=Fixed-point  arith_type=Unsigned  n_bits=outputs  bin_pt=0  preci_type=Single  exp_width=8  frac_width=24  explicit_period=off  period=1  equ=P=C  opselect=C  inp2=PCIN>>17  opr=+  inp1=P  carry=CIN  dbl_ovrd=off  block_type=constant
  Constant4 : xbsIndex_r4/Constant  const=2^(period-outputs-1)-delay  gui_display_data_type=Fixed-point  arith_type=Signed (2's comp)  n_bits=period-outputs  bin_pt=0  preci_type=Single  exp_width=8  frac_width=24  explicit_period=off  period=1  equ=P=C  opselect=C  inp2=PCIN>>17  opr=+  inp1=P  carry=CIN  dbl_ovrd=off  block_type=constant
  Constant5 : xbsIndex_r4/Constant  const=4  gui_display_data_type=Fixed-point  arith_type=Unsigned  n_bits=outputs  bin_pt=0  preci_type=Single  exp_width=8  frac_width=24  explicit_period=off  period=1  equ=P=C  opselect=C  inp2=PCIN>>17  opr=+  inp1=P  carry=CIN  dbl_ovrd=off  block_type=constant
  Constant6 : xbsIndex_r4/Constant  const=5  gui_display_data_type=Fixed-point  arith_type=Unsigned  n_bits=outputs  bin_pt=0  preci_type=Single  exp_width=8  frac_width=24  explicit_period=off  period=1  equ=P=C  opselect=C  inp2=PCIN>>17  opr=+  inp1=P  carry=CIN  dbl_ovrd=off  block_type=constant
  Constant7 : xbsIndex_r4/Constant  const=6  gui_display_data_type=Fixed-point  arith_type=Unsigned  n_bits=outputs  bin_pt=0  preci_type=Single  exp_width=8  frac_width=24  explicit_period=off  period=1  equ=P=C  opselect=C  inp2=PCIN>>17  opr=+  inp1=P  carry=CIN  dbl_ovrd=off  block_type=constant
  Constant8 : xbsIndex_r4/Constant  const=7  gui_display_data_type=Fixed-point  arith_type=Unsigned  n_bits=outputs  bin_pt=0  preci_type=Single  exp_width=8  frac_width=24  explicit_period=off  period=1  equ=P=C  opselect=C  inp2=PCIN>>17  opr=+  inp1=P  carry=CIN  dbl_ovrd=off  block_type=constant
  Counter : xbsIndex_r4/Counter  cnt_type=Free Running  cnt_to=Inf  operation=Up  start_count=-2^(period-outputs-1)  cnt_by_val=1  arith_type="Signed  (2's comp)"  n_bits=period-outputs  bin_pt=0  load_pin=off  rst=on  en=off  explicit_period=on  period=1  dbl_ovrd=off  use_behavioral_HDL=off  implementation=Fabric  use_rpm=off  block_type=counter
  Reinterpret{,1,4,6,8,10,12,14} (8 alike) : xbsIndex_r4/Reinterpret  force_arith_type=on  arith_type=Unsigned  force_bin_pt=on  bin_pt=0  block_type=reinterpret
      settings: infoedit="Changes signal type without altering the binary representation.   You can changed the signal between signed and unsigned, and relocate the binary point.<br><br>Hardware notes: In hardware this block costs nothing.<br><br>Example:  Suppose the input is 6 bits wide, signed, with 2 fractional bits, and the output is forced to unsigned with 0 fractional bits.  Then an input of -2.0 (1110.00 in binary 2's complement) becomes an output of 56 (111000 in binary)."
  Reinterpret{2..3,5,7,9,11,13,15} (8 alike) : xbsIndex_r4/Reinterpret  force_arith_type=on  arith_type="Signed  (2's comp)"  force_bin_pt=on  bin_pt=0  block_type=reinterpret
      settings: infoedit="Changes signal type without altering the binary representation.   You can changed the signal between signed and unsigned, and relocate the binary point.<br><br>Hardware notes: In hardware this block costs nothing.<br><br>Example:  Suppose the input is 6 bits wide, signed, with 2 fractional bits, and the output is forced to unsigned with 0 fractional bits.  Then an input of -2.0 (1110.00 in binary 2's complement) becomes an output of 56 (111000 in binary)."
  Relational : xbsIndex_r4/Relational  mode=a=b  en=off  latency=1  dbl_ovrd=off  block_type=relational
      settings: block_version=10.1.3
  x : Outport
  x+1 : Outport  Port=2
  x+2 : Outport  Port=3
  x+3 : Outport  Port=4
  x+4 : Outport  Port=5
  x+5 : Outport  Port=6
  x+6 : Outport  Port=7
  x+7 : Outport  Port=8
  update : Outport  Port=9
  wires:
  Relational/1 -> update/1
  Constant4/1 -> Relational/2
  Concat1/1 -> Reinterpret3/1
  Constant1/1 -> Concat1/2
  Concat/1 -> Reinterpret2/1
  Constant/1 -> Concat/2
  Counter/1 -> Reinterpret/1, Relational/1, Reinterpret1/1, Reinterpret4/1, Reinterpret6/1, Reinterpret8/1, Reinterpret10/1, Reinterpret12/1, Reinterpret14/1
  sync_in/1 -> Counter/1
  Reinterpret/1 -> Concat/1
  Reinterpret1/1 -> Concat1/1
  Reinterpret2/1 -> x/1
  Reinterpret3/1 -> x+1/1
  Concat2/1 -> Reinterpret5/1
  Constant2/1 -> Concat2/2
  Reinterpret4/1 -> Concat2/1
  Reinterpret5/1 -> x+2/1
  Concat3/1 -> Reinterpret7/1
  Constant3/1 -> Concat3/2
  Reinterpret6/1 -> Concat3/1
  Reinterpret7/1 -> x+3/1
  Concat4/1 -> Reinterpret9/1
  Constant5/1 -> Concat4/2
  Reinterpret8/1 -> Concat4/1
  Reinterpret9/1 -> x+4/1
  Concat5/1 -> Reinterpret11/1
  Constant6/1 -> Concat5/2
  Reinterpret10/1 -> Concat5/1
  Reinterpret11/1 -> x+5/1
  Concat6/1 -> Reinterpret13/1
  Constant7/1 -> Concat6/2
  Reinterpret12/1 -> Concat6/1
  Reinterpret13/1 -> x+6/1
  Concat7/1 -> Reinterpret15/1
  Constant8/1 -> Concat7/2
  Reinterpret14/1 -> Concat7/1
  Reinterpret15/1 -> x+7/1

== system fine_delay_core/fd_fs0/delay_gen0/delay_calc ==
  val : Inport
  val_inc : Inport  Port=2
  en : Inport  Port=3
  update : Inport  Port=4
  AddSub : xbsIndex_r4/AddSub  mode=Addition  use_carryin=off  use_carryout=off  en=off  latency=2  precision=User Defined  arith_type=Unsigned  n_bits=bit_width  bin_pt=bin_pt  quantization=Truncate  overflow=Saturate  dbl_ovrd=off  use_behavioral_HDL=off  hw_selection=DSP48  pipelined=on  use_rpm=on  block_type=addsub
      settings: block_version=10.1.3
  Delay : xbsIndex_r4/Delay  rst=off  infoeditControl=Selection of Reset will increase slice count due to use of real FFs and instead of SRLs  en=off  latency=1  dbl_ovrd=off  reg_retiming=on  block_type=delay
  Delay1 : xbsIndex_r4/Delay  rst=off  infoeditControl=Selection of Reset will increase slice count due to use of real FFs and instead of SRLs  en=off  latency=1  dbl_ovrd=off  reg_retiming=on  block_type=delay
  Gateway Out{,1,3..4} (4 alike) : xbsIndex_r4/Gateway Out  inherit_from_input=off  hdl_port=off  timing_constraint=None  locs_specified=off  LOCs={}  UseAsDAC=off  DACChannel='1'  block_type=gatewayout
      settings: infoedit="Gateway out block.  Converts Xilinx fixed point inputs into ouputs of type Simulink integer, double, or fixed point.<br><br>Hardware notes:  In hardware these blocks become top level output ports or are discarded, depending on how they are configured."  block_version=11.4
  Logical : xbsIndex_r4/Logical  logical_function=OR  inputs=2  en=off  latency=0  precision=Full  arith_type=Unsigned  n_bits=16  bin_pt=0  align_bp=on  dbl_ovrd=off  block_type=logical
  Mux : xbsIndex_r4/Mux  inputs=2  en=off  latency=1  precision=Full  arith_type=Unsigned  n_bits=16  bin_pt=14  quantization=Truncate  overflow=Wrap  dbl_ovrd=off  block_type=mux
  Register : xbsIndex_r4/Register  init=0  rst=on  en=on  dbl_ovrd=off  block_type=register
  Register1 : xbsIndex_r4/Register  init=0  rst=off  en=on  dbl_ovrd=off  block_type=register
  Register3 : xbsIndex_r4/Register  init=0  rst=off  en=on  dbl_ovrd=off  block_type=register
      settings: block_version=11.4
  Scope : Scope  NumInputPorts=4
      settings: YMin=-5~-5~-5~-5  YMax=5~5~5~5  SaveName=ScopeData4
  current : xbsIndex_r4/Register  init=0  rst=off  en=on  dbl_ovrd=off  block_type=register
  delta : xbsIndex_r4/Register  init=0  rst=off  en=on  dbl_ovrd=off  block_type=register
  coeff : Outport
  en_o : Outport  Port=2
  wires:
  Register1/1 -> delta/1
  val_inc/1 -> Register1/1
  AddSub/1 -> Mux/2
  Register3/1 -> Mux/3
  val/1 -> Register3/1
  Gateway Out1/1 -> Scope/4
  Gateway Out4/1 -> Scope/3
  Gateway Out3/1 -> Scope/2
  Gateway Out/1 -> Scope/1
  current/1 -> coeff/1, AddSub/1
  delta/1 -> Gateway Out1/1, AddSub/2
  Mux/1 -> Gateway Out/1, current/1
  en/1 -> Register1/2, Register3/2, Register/3, Gateway Out4/1, Logical/1, Register/1
  update/1 -> Gateway Out3/1, Delay/1, Register/2
  Register/1 -> Logical/2
  Logical/1 -> Mux/1
  Delay/1 -> delta/2, current/2, Delay1/1
  Delay1/1 -> en_o/1

== system fine_delay_core/fd_fs0/delay_gen0/phase_calc ==
  val : Inport
  val_inc : Inport  Port=2
  en : Inport  Port=3
  update : Inport  Port=4
  AddSub : xbsIndex_r4/AddSub  mode=Addition  use_carryin=off  use_carryout=off  en=off  latency=2  precision=User Defined  arith_type="Signed  (2's comp)"  n_bits=bit_width  bin_pt=bin_pt  quantization=Truncate  overflow=Wrap  dbl_ovrd=off  use_behavioral_HDL=off  hw_selection=DSP48  pipelined=on  use_rpm=on  block_type=addsub
      settings: block_version=10.1.3
  Delay : xbsIndex_r4/Delay  rst=off  infoeditControl=Selection of Reset will increase slice count due to use of real FFs and instead of SRLs  en=off  latency=1  dbl_ovrd=off  reg_retiming=on  block_type=delay
  Delay1 : xbsIndex_r4/Delay  rst=off  infoeditControl=Selection of Reset will increase slice count due to use of real FFs and instead of SRLs  en=off  latency=1  dbl_ovrd=off  reg_retiming=on  block_type=delay
  Gateway Out{,1,3..4} (4 alike) : xbsIndex_r4/Gateway Out  inherit_from_input=off  hdl_port=off  timing_constraint=None  locs_specified=off  LOCs={}  UseAsDAC=off  DACChannel='1'  block_type=gatewayout
      settings: infoedit="Gateway out block.  Converts Xilinx fixed point inputs into ouputs of type Simulink integer, double, or fixed point.<br><br>Hardware notes:  In hardware these blocks become top level output ports or are discarded, depending on how they are configured."  block_version=11.4
  Logical : xbsIndex_r4/Logical  logical_function=OR  inputs=2  en=off  latency=0  precision=Full  arith_type=Unsigned  n_bits=16  bin_pt=0  align_bp=on  dbl_ovrd=off  block_type=logical
  Mux : xbsIndex_r4/Mux  inputs=2  en=off  latency=1  precision=Full  arith_type=Unsigned  n_bits=16  bin_pt=14  quantization=Truncate  overflow=Wrap  dbl_ovrd=off  block_type=mux
  Register : xbsIndex_r4/Register  init=0  rst=on  en=on  dbl_ovrd=off  block_type=register
  Register1 : xbsIndex_r4/Register  init=0  rst=off  en=on  dbl_ovrd=off  block_type=register
  Register3 : xbsIndex_r4/Register  init=0  rst=off  en=on  dbl_ovrd=off  block_type=register
      settings: block_version=11.4
  Scope : Scope  NumInputPorts=4
      settings: YMin=-5~-5~-5~-5  YMax=5~5~5~5  SaveName=ScopeData4
  current : xbsIndex_r4/Register  init=0  rst=off  en=on  dbl_ovrd=off  block_type=register
  delta : xbsIndex_r4/Register  init=0  rst=off  en=on  dbl_ovrd=off  block_type=register
  coeff : Outport
  en_o : Outport  Port=2
  wires:
  Delay1/1 -> en_o/1
  Delay/1 -> Delay1/1, current/2, delta/2
  Logical/1 -> Mux/1
  Register/1 -> Logical/2
  update/1 -> Register/2, Delay/1, Gateway Out3/1
  en/1 -> Register/1, Logical/1, Gateway Out4/1, Register/3, Register3/2, Register1/2
  Mux/1 -> current/1, Gateway Out/1
  delta/1 -> AddSub/2, Gateway Out1/1
  current/1 -> AddSub/1, coeff/1
  Gateway Out/1 -> Scope/1
  Gateway Out3/1 -> Scope/2
  Gateway Out4/1 -> Scope/3
  Gateway Out1/1 -> Scope/4
  val/1 -> Register3/1
  Register3/1 -> Mux/3
  AddSub/1 -> Mux/2
  val_inc/1 -> Register1/1
  Register1/1 -> delta/1

== system fine_delay_core/fd_fs0/fd_fs0/bus2_0 ==
  in1 : Inport
  in2 : Inport  Port=2
  in3 : Inport  Port=3
  in4 : Inport  Port=4
  in5 : Inport  Port=5
  in6 : Inport  Port=6
  in7 : Inport  Port=7
  in8 : Inport  Port=8
  concatenate : xbsIndex_r4/Concat  num_inputs=8  dbl_ovrd=off  block_type=concat
  reinterpret{1..8} (8 alike) : xbsIndex_r4/Reinterpret  force_arith_type=on  arith_type=Unsigned  force_bin_pt=on  bin_pt=0  block_type=reinterpret
      reinterpret1 settings: infoedit="Changes signal type without altering the binary representation.   You can changed the signal between signed and unsigned, and relocate the binary point.<br><br>Hardware notes: In hardware this block costs nothing.<br><br>Example:  Suppose the input is 6 bits wide, signed, with 2 fractional bits, and the output is forced to unsigned with 0 fractional bits.  Then an input of -2.0 (1110.00 in binary 2's complement) becomes an output of 56 (111000 in binary)."
      reinterpret2 settings: infoedit="Changes signal type without altering the binary representation.   You can changed the signal between signed and unsigned, and relocate the binary point.<br><br>Hardware notes: In hardware this block costs nothing.<br><br>Example:  Suppose the input is 6 bits wide, signed, with 2 fractional bits, and the output is forced to unsigned with 0 fractional bits.  Then an input of -2.0 (1110.00 in binary 2's complement) becomes an output of 56 (111000 in binary)."
  bus_out : Outport
  wires:
  concatenate/1 -> bus_out/1
  in1/1 -> reinterpret1/1
  reinterpret1/1 -> concatenate/1
  in2/1 -> reinterpret2/1
  reinterpret2/1 -> concatenate/2
  in3/1 -> reinterpret3/1
  reinterpret3/1 -> concatenate/3
  in4/1 -> reinterpret4/1
  reinterpret4/1 -> concatenate/4
  in5/1 -> reinterpret5/1
  reinterpret5/1 -> concatenate/5
  in6/1 -> reinterpret6/1
  reinterpret6/1 -> concatenate/6
  in7/1 -> reinterpret7/1
  reinterpret7/1 -> concatenate/7
  in8/1 -> reinterpret8/1
  reinterpret8/1 -> concatenate/8
